simulink model "wrapper_exp"  (R2018a)
settings: Solver=FixedStepAuto  StartTime=0.0  StopTime=120  FixedStep=0.05  MaxStep=0.5  MinStep=0.3  RelTol=10  AbsTol=10
model workspace (MAT data in the model file):
  SL_ROS_VariableLengthArrays_MaxSizes.CommonInfo.ArrayTruncateAction = 'EmitWarning'
  SL_ROS_VariableLengthArrays_MaxSizes.MsgTypeMap = containers.Map
  SL_ROS_VariableLengthArrays_MaxSizes.MsgTypeMap.serialization.keys = {'sensor_msgs/CompressedImage', 'sensor_msgs/Image'}
  SL_ROS_VariableLengthArrays_MaxSizes.MsgTypeMap.serialization.values{1}(1).PropertyName = 'Data'
  SL_ROS_VariableLengthArrays_MaxSizes.MsgTypeMap.serialization.values{1}(1).DataType = 'uint8'
  SL_ROS_VariableLengthArrays_MaxSizes.MsgTypeMap.serialization.values{1}(1).MaxLength = 200000
  SL_ROS_VariableLengthArrays_MaxSizes.MsgTypeMap.serialization.values{1}(2).PropertyName = 'Format'
  SL_ROS_VariableLengthArrays_MaxSizes.MsgTypeMap.serialization.values{1}(2).DataType = 'uint8'
  SL_ROS_VariableLengthArrays_MaxSizes.MsgTypeMap.serialization.values{1}(2).MaxLength = 128
  SL_ROS_VariableLengthArrays_MaxSizes.MsgTypeMap.serialization.values{2}(1).PropertyName = 'Data'
  SL_ROS_VariableLengthArrays_MaxSizes.MsgTypeMap.serialization.values{2}(1).DataType = 'uint8'
  SL_ROS_VariableLengthArrays_MaxSizes.MsgTypeMap.serialization.values{2}(1).MaxLength = 2764800
  SL_ROS_VariableLengthArrays_MaxSizes.MsgTypeMap.serialization.values{2}(2).PropertyName = 'Encoding'
  SL_ROS_VariableLengthArrays_MaxSizes.MsgTypeMap.serialization.values{2}(2).DataType = 'uint8'
  SL_ROS_VariableLengthArrays_MaxSizes.MsgTypeMap.serialization.values{2}(2).MaxLength = 128
  SL_ROS_VariableLengthArrays_MaxSizes.MsgTypeMap.serialization.uniformity = 0
  SL_ROS_VariableLengthArrays_MaxSizes.MsgTypeMap.serialization.keyType = 'char'
  SL_ROS_VariableLengthArrays_MaxSizes.MsgTypeMap.serialization.valueType = 'any'
undefined symbols (not defined in the file or in its folder): Angular, Linear
libraries: robotlib x12, sharedtransform x2, aerolibutil x1, vrlib x1
settings Model: EnablePacing=on  Creator=lenny  LastModifiedBy=lenny
settings SolverCC: MaxConsecutiveMinStep=99999  ShapePreserveControl=EnableAll

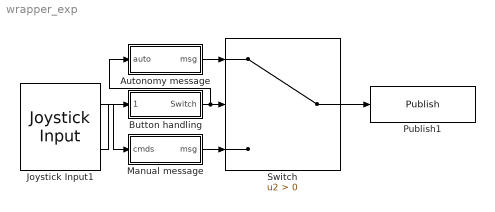
== system wrapper_exp ==
  Autonomy message : Subsystem
  Button handling : Subsystem
  Joystick Input1 : vrlib/Joystick Input  joyid=1  adjustports=on  forcefeed=off
      settings: SourceProductBaseCode=VR
  Manual message : Subsystem
  Publish1 : robotlib/Publish  SourceLibraryInfo=This block requires Robotics System Toolbox  topicSource=Specify your own  topic=/auto/cmd  messageType=geometry_msgs/Twist  messageQueueLength=1
      settings: SourceProductBaseCode=RO
  Switch : Switch  Criteria=u2 > Threshold
  wires:
  Joystick Input1/1 -> Manual message/1(cmds)
  Switch/1 -> Publish1/1
  Autonomy message/1(msg) -> Switch/1
  Manual message/1(msg) -> Switch/3
  Joystick Input1/2 -> Button handling/1(Buttons)
  Button handling/1(Switch) -> Autonomy message/1(auto), Switch/2

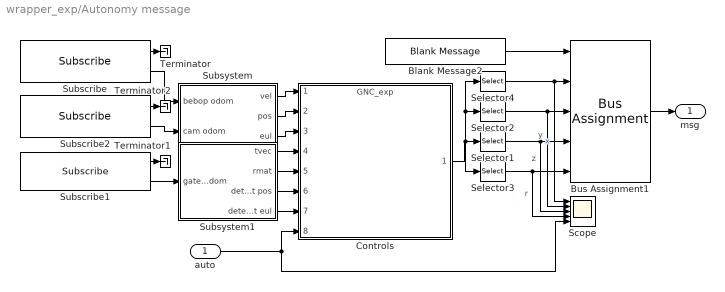
== system wrapper_exp/Autonomy message ==
  auto : Inport
  Blank Message2 : robotlib/Blank Message  SourceLibraryInfo=This block requires Robotics System Toolbox  messageType=geometry_msgs/Twist  SampleTime=inf
      settings: SourceProductBaseCode=RO
  Bus Assignment1 : BusAssignment  AssignedSignals=Linear.X,Linear.Y,Linear.Z,Angular.Z
  Controls : ModelReference  ModelNameDialog=GNC_exp.slx  SimulationMode=Normal  ModelReferenceVersion=1.498
  Scope : Scope  NumInputPorts=5
  Selector1 : Selector  InputPortWidth=4  IndexOptions=Index vector (dialog)  Indices=3  OutputSizes=1
  Selector2 : Selector  InputPortWidth=4  IndexOptions=Index vector (dialog)  Indices=2  OutputSizes=1
  Selector3 : Selector  InputPortWidth=4  IndexOptions=Index vector (dialog)  Indices=4  OutputSizes=1
  Selector4 : Selector  InputPortWidth=4  IndexOptions=Index vector (dialog)  Indices=1  OutputSizes=1
  Subscribe : robotlib/Subscribe  SourceLibraryInfo=This block requires Robotics System Toolbox  topicSource=Select from ROS network  topic=/bebop/odom  messageType=nav_msgs/Odometry  sampleTime=-1  messageQueueLength=1
      settings: SourceProductBaseCode=RO
  Subscribe1 : robotlib/Subscribe  SourceLibraryInfo=This block requires Robotics System Toolbox  topicSource=Select from ROS network  topic=/auto/gate_detection_Odom  messageType=nav_msgs/Odometry  sampleTime=-1  messageQueueLength=1
      settings: SourceProductBaseCode=RO
  Subscribe2 : robotlib/Subscribe  SourceLibraryInfo=This block requires Robotics System Toolbox  topicSource=Select from ROS network  topic=/zed/odom  messageType=nav_msgs/Odometry  sampleTime=-1  messageQueueLength=1
      settings: SourceProductBaseCode=RO
  Subsystem : Subsystem
  Subsystem1 : Subsystem
  Terminator : Terminator
  Terminator1 : Terminator
  Terminator2 : Terminator
  msg : Outport
  wires:
  Selector2/1 -> Scope/2, Bus Assignment1/3  "y"
  Subscribe1/1 -> Terminator1/1
  Bus Assignment1/1 -> msg/1
  Selector4/1 -> Scope/1, Bus Assignment1/2  "x"
  Subscribe1/2 -> Subsystem1/1(gateOdom)
  Subscribe/2 -> Subsystem/1(bebop odom)
  Subsystem/2(pos) -> Controls/2
  Subsystem1/1(tvec) -> Controls/4
  Subscribe/1 -> Terminator/1
  Selector3/1 -> Scope/4, Bus Assignment1/5  "r"
  Blank Message2/1 -> Bus Assignment1/1
  Subsystem/1(vel) -> Controls/1
  Controls/1 -> Selector4/1, Selector2/1, Selector3/1, Selector1/1
  Subsystem/3(eul) -> Controls/3
  Selector1/1 -> Scope/3, Bus Assignment1/4  "z"
  auto/1 -> Scope/5, Controls/8
  Subsystem1/2(rmat) -> Controls/5
  Subsystem1/3(detect pos) -> Controls/6
  Subsystem1/4(detect eul) -> Controls/7
  Subscribe2/1 -> Terminator2/1
  Subscribe2/2 -> Subsystem/2(cam odom)

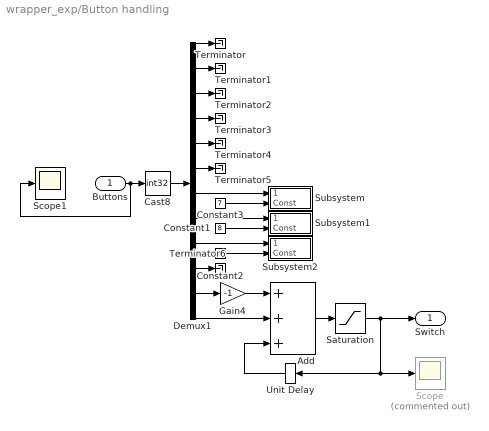
== system wrapper_exp/Button handling ==
  Buttons : Inport
  Add : Sum  Inputs=+++
  Cast8 : DataTypeConversion  OutDataTypeStr=int32
  Constant1 : Constant  Value=8
  Constant2 : Constant  Value=9
  Constant3 : Constant  Value=7
  Demux1 : Demux  Outputs=12
  Gain4 : Gain  Gain=-1
  Saturation : Saturate  UpperLimit=1  LowerLimit=0
  Scope : Scope  Commented=on
  Scope1 : Scope
  Subsystem : Subsystem
  Subsystem1 : Subsystem
  Subsystem2 : Subsystem
  Terminator{,1..6} (7 alike) : Terminator
  Unit Delay : UnitDelay  SampleTime=-1
  Switch : Outport
  wires:
  Demux1/2 -> Terminator1/1
  Demux1/6 -> Terminator5/1
  Constant1/1 -> Subsystem1/2(Const)
  Demux1/3 -> Terminator2/1
  Demux1/8 -> Subsystem1/1(Button)
  Demux1/9 -> Subsystem2/1(Button)
  Demux1/12 -> Add/2
  Constant2/1 -> Subsystem2/2(Const)
  Add/1 -> Saturation/1
  Cast8/1 -> Demux1/1
  Demux1/7 -> Subsystem/1(Button)
  Saturation/1 -> Scope/1, Unit Delay/1, Switch/1
  Unit Delay/1 -> Add/3
  Buttons/1 -> Scope1/1, Cast8/1
  Demux1/4 -> Terminator3/1
  Demux1/1 -> Terminator/1
  Demux1/5 -> Terminator4/1
  Demux1/11 -> Gain4/1
  Constant3/1 -> Subsystem/2(Const)
  Demux1/10 -> Terminator6/1
  Gain4/1 -> Add/1

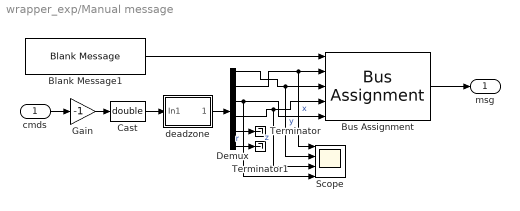
== system wrapper_exp/Manual message ==
  cmds : Inport
  Blank Message1 : robotlib/Blank Message  SourceLibraryInfo=This block requires Robotics System Toolbox  messageType=geometry_msgs/Twist  SampleTime=inf
      settings: SourceProductBaseCode=RO
  Bus Assignment : BusAssignment  AssignedSignals=Linear.X,Linear.Y,Linear.Z,Angular.Z
  Cast : DataTypeConversion  OutDataTypeStr=double
  Demux : Demux  Outputs=6
  Gain : Gain  Gain=-1
  Scope : Scope  NumInputPorts=4
  Terminator : Terminator
  Terminator1 : Terminator
  deadzone : Subsystem
  msg : Outport
  wires:
  Demux/2 -> Scope/1, Bus Assignment/2  "x"
  Demux/4 -> Scope/3, Bus Assignment/4  "z"
  Demux/6 -> Terminator1/1
  Blank Message1/1 -> Bus Assignment/1
  Demux/1 -> Scope/2, Bus Assignment/3  "y"
  cmds/1 -> Gain/1
  Demux/3 -> Bus Assignment/5, Scope/4  "r"
  Bus Assignment/1 -> msg/1
  Demux/5 -> Terminator/1
  Cast/1 -> deadzone/1(In1)
  Gain/1 -> Cast/1
  deadzone/1(Out1) -> Demux/1

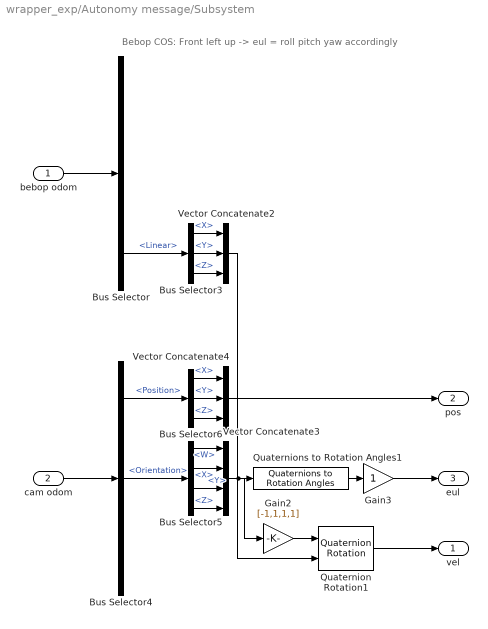
== system wrapper_exp/Autonomy message/Subsystem ==
  note: Bebop COS: Front left up -> eul = roll pitch yaw accordingly
  bebop odom : Inport
  cam odom : Inport  Port=2
  Bus Selector : BusSelector  OutputSignals=Pose.Pose.Position,Pose.Pose.Orientation,Twist.Twist.Linear
  Bus Selector3 : BusSelector  OutputSignals=X,Y,Z
  Bus Selector4 : BusSelector  OutputSignals=Pose.Pose.Position,Pose.Pose.Orientation,Twist.Twist.Linear
  Bus Selector5 : BusSelector  OutputSignals=W,X,Y,Z
  Bus Selector6 : BusSelector  OutputSignals=X,Y,Z
  Gain2 : Gain  Gain=[-1,1,1,1]
  Gain3 : Gain
  Quaternion Rotation1 : aerolibutil/Quaternion Rotation
  Quaternions to Rotation Angles1 : sharedtransform/Quaternions to Rotation Angles  rotationOrder=XYZ  aMode=aMode
      settings: SourceProductBaseCode=AE
  Vector Concatenate2 : Concatenate  NumInputs=3
  Vector Concatenate3 : Concatenate  NumInputs=4
  Vector Concatenate4 : Concatenate  NumInputs=3
  vel : Outport
  pos : Outport  Port=2
  eul : Outport  Port=3
  wires:
  bebop odom/1 -> Bus Selector/1
  Bus Selector/3 -> Bus Selector3/1  "<Linear>"
  Bus Selector3/2 -> Vector Concatenate2/2  "<Y>"
  Bus Selector3/1 -> Vector Concatenate2/1  "<X>"
  Bus Selector3/3 -> Vector Concatenate2/3  "<Z>"
  Bus Selector6/3 -> Vector Concatenate4/3  "<Z>"
  Bus Selector4/1 -> Bus Selector6/1  "<Position>"
  Gain2/1 -> Quaternion Rotation1/1
  Bus Selector6/1 -> Vector Concatenate4/1  "<X>"
  Bus Selector5/1 -> Vector Concatenate3/1  "<W>"
  Vector Concatenate3/1 -> Gain2/1, Quaternions to Rotation Angles1/1
  Bus Selector5/4 -> Vector Concatenate3/4  "<Z>"
  Bus Selector5/2 -> Vector Concatenate3/2  "<X>"
  cam odom/1 -> Bus Selector4/1
  Vector Concatenate2/1 -> Quaternion Rotation1/2
  Bus Selector4/2 -> Bus Selector5/1  "<Orientation>"
  Quaternions to Rotation Angles1/1 -> Gain3/1
  Bus Selector6/2 -> Vector Concatenate4/2  "<Y>"
  Bus Selector5/3 -> Vector Concatenate3/3  "<Y>"
  Vector Concatenate4/1 -> pos/1
  Gain3/1 -> eul/1
  Quaternion Rotation1/1 -> vel/1

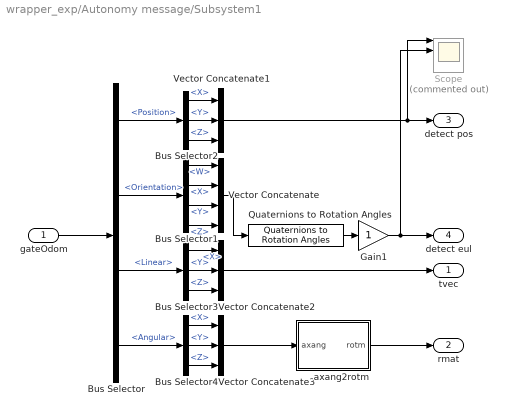
== system wrapper_exp/Autonomy message/Subsystem1 ==
  gateOdom : Inport
  Bus Selector : BusSelector  OutputSignals=Pose.Pose.Position,Pose.Pose.Orientation,Twist.Twist.Linear,Twist.Twist.Angular
  Bus Selector1 : BusSelector  OutputSignals=W,X,Y,Z
  Bus Selector2 : BusSelector  OutputSignals=X,Y,Z
  Bus Selector3 : BusSelector  OutputSignals=X,Y,Z
  Bus Selector4 : BusSelector  OutputSignals=X,Y,Z
  Gain1 : Gain
  Quaternions to Rotation Angles : sharedtransform/Quaternions to Rotation Angles  rotationOrder=XYZ  aMode=aMode
      settings: SourceProductBaseCode=AE
  Scope : Scope  Commented=on  NumInputPorts=4
  Vector Concatenate : Concatenate  NumInputs=4
  Vector Concatenate1 : Concatenate  NumInputs=3
  Vector Concatenate2 : Concatenate  NumInputs=3  Mode=Multidimensional array
  Vector Concatenate3 : Concatenate  NumInputs=3
  axang2rotm : MATLAB Function  TreatAsAtomicUnit=on
  tvec : Outport
  rmat : Outport  Port=2
  detect pos : Outport  Port=3
  detect eul : Outport  Port=4
  wires:
  Bus Selector/1 -> Bus Selector2/1  "<Position>"
  Gain1/1 -> Scope/2, detect eul/1
  gateOdom/1 -> Bus Selector/1
  Bus Selector/2 -> Bus Selector1/1  "<Orientation>"
  Bus Selector1/1 -> Vector Concatenate/1  "<W>"
  Bus Selector1/2 -> Vector Concatenate/2  "<X>"
  Bus Selector1/3 -> Vector Concatenate/3  "<Y>"
  Bus Selector1/4 -> Vector Concatenate/4  "<Z>"
  Vector Concatenate/1 -> Quaternions to Rotation Angles/1
  Bus Selector2/2 -> Vector Concatenate1/2  "<Y>"
  Bus Selector2/1 -> Vector Concatenate1/1  "<X>"
  Bus Selector2/3 -> Vector Concatenate1/3  "<Z>"
  Vector Concatenate1/1 -> Scope/1, detect pos/1
  Bus Selector/3 -> Bus Selector3/1  "<Linear>"
  Bus Selector3/2 -> Vector Concatenate2/2  "<Y>"
  Bus Selector3/1 -> Vector Concatenate2/1  "<X>"
  Bus Selector3/3 -> Vector Concatenate2/3  "<Z>"
  Quaternions to Rotation Angles/1 -> Gain1/1
  Bus Selector/4 -> Bus Selector4/1  "<Angular>"
  Bus Selector4/1 -> Vector Concatenate3/1  "<X>"
  Bus Selector4/2 -> Vector Concatenate3/2  "<Y>"
  Bus Selector4/3 -> Vector Concatenate3/3  "<Z>"
  Vector Concatenate3/1 -> axang2rotm/1(axang)
  Vector Concatenate2/1 -> tvec/1
  axang2rotm/1(rotm) -> rmat/1

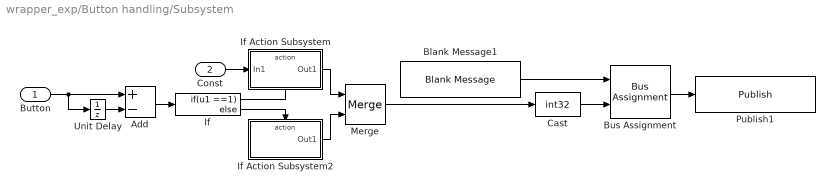
== system wrapper_exp/Button handling/Subsystem ==
  Button : Inport
  Const : Inport  Port=2
  Add : Sum  Inputs=+-
  Blank Message1 : robotlib/Blank Message  SourceLibraryInfo=This block requires Robotics System Toolbox  messageType=std_msgs/Int32  SampleTime=inf
      settings: SourceProductBaseCode=RO
  Bus Assignment : BusAssignment  AssignedSignals=Data
  Cast : DataTypeConversion  OutDataTypeStr=int32
  If : If  IfExpression=u1 ==1
  If Action Subsystem : Subsystem  TreatAsAtomicUnit=on
  If Action Subsystem2 : Subsystem  TreatAsAtomicUnit=on
  Merge : Merge
  Publish1 : robotlib/Publish  SourceLibraryInfo=This block requires Robotics System Toolbox  topicSource=Specify your own  topic=/auto/flt_st_cmd  messageType=std_msgs/Int32  messageQueueLength=1
      settings: SourceProductBaseCode=RO
  Unit Delay : UnitDelay  SampleTime=-1
  wires:
  If Action Subsystem/1(Out1) -> Merge/1
  Add/1 -> If/1
  Button/1 -> Unit Delay/1, Add/1
  Cast/1 -> Bus Assignment/2
  If/1 -> If Action Subsystem/Action
  If Action Subsystem2/1(Out1) -> Merge/2
  If/2 -> If Action Subsystem2/Action
  Bus Assignment/1 -> Publish1/1
  Blank Message1/1 -> Bus Assignment/1
  Unit Delay/1 -> Add/2
  Const/1 -> If Action Subsystem/1(In1)
  Merge/1 -> Cast/1

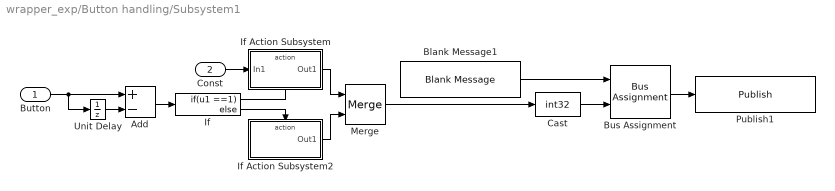
== system wrapper_exp/Button handling/Subsystem1 ==
  Button : Inport
  Const : Inport  Port=2
  Add : Sum  Inputs=+-
  Blank Message1 : robotlib/Blank Message  SourceLibraryInfo=This block requires Robotics System Toolbox  messageType=std_msgs/Int32  SampleTime=inf
      settings: SourceProductBaseCode=RO
  Bus Assignment : BusAssignment  AssignedSignals=Data
  Cast : DataTypeConversion  OutDataTypeStr=int32
  If : If  IfExpression=u1 ==1
  If Action Subsystem : Subsystem  TreatAsAtomicUnit=on
  If Action Subsystem2 : Subsystem  TreatAsAtomicUnit=on
  Merge : Merge
  Publish1 : robotlib/Publish  SourceLibraryInfo=This block requires Robotics System Toolbox  topicSource=Specify your own  topic=/auto/flt_st_cmd  messageType=std_msgs/Int32  messageQueueLength=1
      settings: SourceProductBaseCode=RO
  Unit Delay : UnitDelay  SampleTime=-1
  wires:
  If Action Subsystem/1(Out1) -> Merge/1
  Add/1 -> If/1
  Button/1 -> Unit Delay/1, Add/1
  Cast/1 -> Bus Assignment/2
  If/1 -> If Action Subsystem/Action
  If Action Subsystem2/1(Out1) -> Merge/2
  If/2 -> If Action Subsystem2/Action
  Bus Assignment/1 -> Publish1/1
  Blank Message1/1 -> Bus Assignment/1
  Unit Delay/1 -> Add/2
  Const/1 -> If Action Subsystem/1(In1)
  Merge/1 -> Cast/1

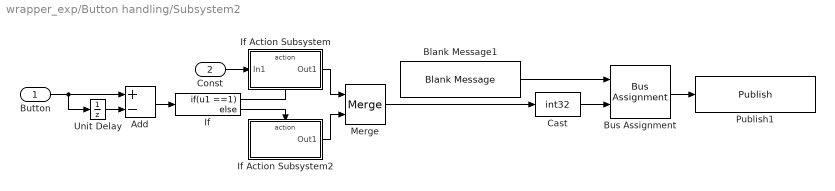
== system wrapper_exp/Button handling/Subsystem2 ==
  Button : Inport
  Const : Inport  Port=2
  Add : Sum  Inputs=+-
  Blank Message1 : robotlib/Blank Message  SourceLibraryInfo=This block requires Robotics System Toolbox  messageType=std_msgs/Int32  SampleTime=inf
      settings: SourceProductBaseCode=RO
  Bus Assignment : BusAssignment  AssignedSignals=Data
  Cast : DataTypeConversion  OutDataTypeStr=int32
  If : If  IfExpression=u1 ==1
  If Action Subsystem : Subsystem  TreatAsAtomicUnit=on
  If Action Subsystem2 : Subsystem  TreatAsAtomicUnit=on
  Merge : Merge
  Publish1 : robotlib/Publish  SourceLibraryInfo=This block requires Robotics System Toolbox  topicSource=Specify your own  topic=/auto/flt_st_cmd  messageType=std_msgs/Int32  messageQueueLength=1
      settings: SourceProductBaseCode=RO
  Unit Delay : UnitDelay  SampleTime=-1
  wires:
  If Action Subsystem/1(Out1) -> Merge/1
  Add/1 -> If/1
  Button/1 -> Unit Delay/1, Add/1
  Cast/1 -> Bus Assignment/2
  If/1 -> If Action Subsystem/Action
  If Action Subsystem2/1(Out1) -> Merge/2
  If/2 -> If Action Subsystem2/Action
  Bus Assignment/1 -> Publish1/1
  Blank Message1/1 -> Bus Assignment/1
  Unit Delay/1 -> Add/2
  Const/1 -> If Action Subsystem/1(In1)
  Merge/1 -> Cast/1

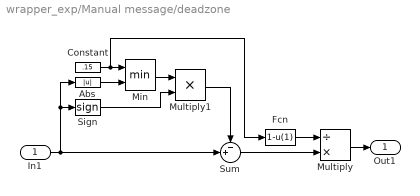
== system wrapper_exp/Manual message/deadzone ==
  In1 : Inport
  Abs : Abs
  Constant : Constant  Value=.15
  Fcn : Fcn  Expr=1-u(1)
  Min : MinMax  Inputs=2
  Multiply : Product  Inputs=/*
  Multiply1 : Product
  Sign : Signum
  Sum : Sum  Inputs=-+|
  Out1 : Outport
  wires:
  In1/1 -> Sum/2, Sign/1, Abs/1
  Constant/1 -> Fcn/1, Min/1
  Min/1 -> Multiply1/1
  Sum/1 -> Multiply/2
  Multiply/1 -> Out1/1
  Abs/1 -> Min/2
  Sign/1 -> Multiply1/2
  Multiply1/1 -> Sum/1
  Fcn/1 -> Multiply/1

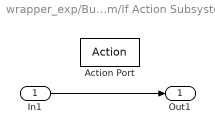
== system wrapper_exp/Button handling/Subsystem/If Action Subsystem ==
  In1 : Inport
  Action Port : ActionPort  ActionType=then
  Out1 : Outport
  wires:
  In1/1 -> Out1/1

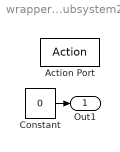
== system wrapper_exp/Button handling/Subsystem/If Action Subsystem2 ==
  Action Port : ActionPort  ActionType=else
  Constant : Constant  Value=0
  Out1 : Outport
  wires:
  Constant/1 -> Out1/1

== system wrapper_exp/Button handling/Subsystem1/If Action Subsystem ==
  In1 : Inport
  Action Port : ActionPort  ActionType=then
  Out1 : Outport
  wires:
  In1/1 -> Out1/1

== system wrapper_exp/Button handling/Subsystem1/If Action Subsystem2 ==
  Action Port : ActionPort  ActionType=else
  Constant : Constant  Value=0
  Out1 : Outport
  wires:
  Constant/1 -> Out1/1

== system wrapper_exp/Button handling/Subsystem2/If Action Subsystem ==
  In1 : Inport
  Action Port : ActionPort  ActionType=then
  Out1 : Outport
  wires:
  In1/1 -> Out1/1

== system wrapper_exp/Button handling/Subsystem2/If Action Subsystem2 ==
  Action Port : ActionPort  ActionType=else
  Constant : Constant  Value=0
  Out1 : Outport
  wires:
  Constant/1 -> Out1/1

== matlab function wrapper_exp/Autonomy message/Subsystem1/axang2rotm ==
  data: axang input; rotm output
function rotm = fcn(axang)
rotm = zeros(3,3);

if ~isequal(axang, zeros(3,1))
    rotm = axang2rotm([axang;norm(axang)]');
end
